simulink model "CTRL_UP_test"  (R2023b)
settings: Solver=VariableStepAuto  StartTime=0.0  StopTime=10.0  RelTol=1e-3
libraries: CTRL_UP x1, simulink x1
settings Model: Creator=blatak  LastModifiedBy=blatak

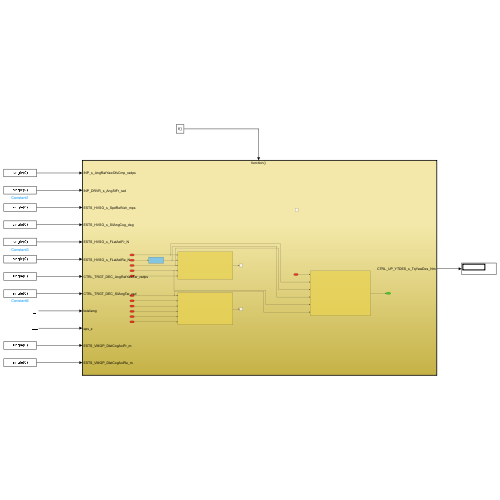
[thumbnail: Simulink's stored preview of the top-level diagram]
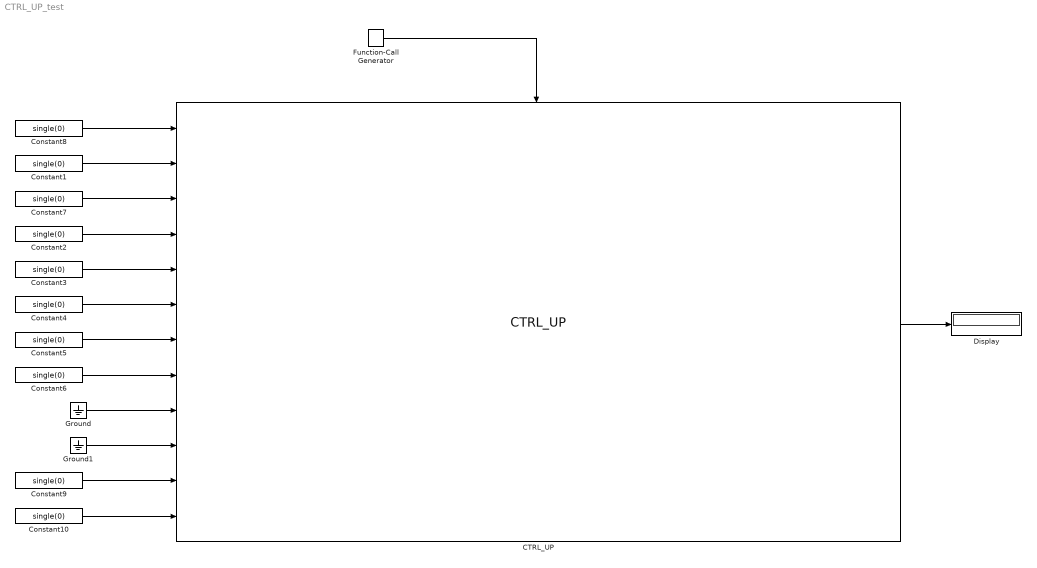
== system CTRL_UP_test ==
  CTRL_UP : CTRL_UP/CTRL_UP  SystemSampleTime=-1  VariantActivationTime=update diagram  AllowFlexibleInterface=on  Latency=0  AutoFrameSizeCalculation=off
  Constant{1..10} (10 alike) : Constant  Value=single(0)  OutDataTypeStr=single
  Display : Display
  Function-Call Generator : simulink/Ports & Subsystems/Function-Call Generator  sample_time=0.01  numberOfIterations=1  DisallowWideOutput=off
  Ground : Ground
  Ground1 : Ground
  wires:
  Function-Call Generator/1 -> CTRL_UP/Trigger
  CTRL_UP/1 -> Display/1
  Constant8/1 -> CTRL_UP/1
  Constant1/1 -> CTRL_UP/2
  Constant7/1 -> CTRL_UP/3
  Constant2/1 -> CTRL_UP/4
  Constant3/1 -> CTRL_UP/5
  Constant4/1 -> CTRL_UP/6
  Constant5/1 -> CTRL_UP/7
  Constant6/1 -> CTRL_UP/8
  Ground/1 -> CTRL_UP/9
  Ground1/1 -> CTRL_UP/10
  Constant9/1 -> CTRL_UP/11
  Constant10/1 -> CTRL_UP/12
